simulink library "TemperatureControlLibrary"  (R2024a)
settings: Solver=VariableStepAuto  StartTime=0.0  StopTime=10.0  RelTol=1e-3
undefined symbols (not defined in the file): delay_s, wn, zetaK
libraries: LumArduinoMAX31856 x1, arduinolib x1
settings Model: Creator=chris  LastModifiedBy=chris

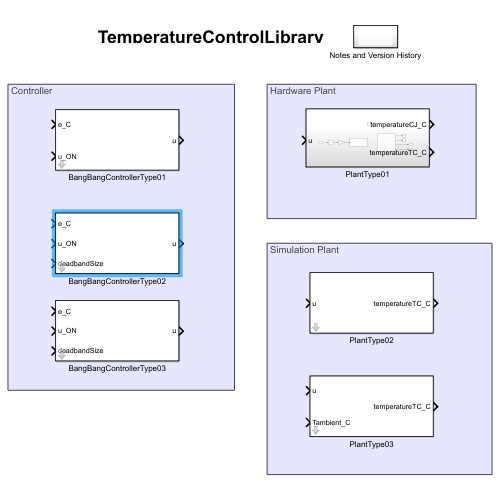
[thumbnail: Simulink's stored preview of the top-level diagram]
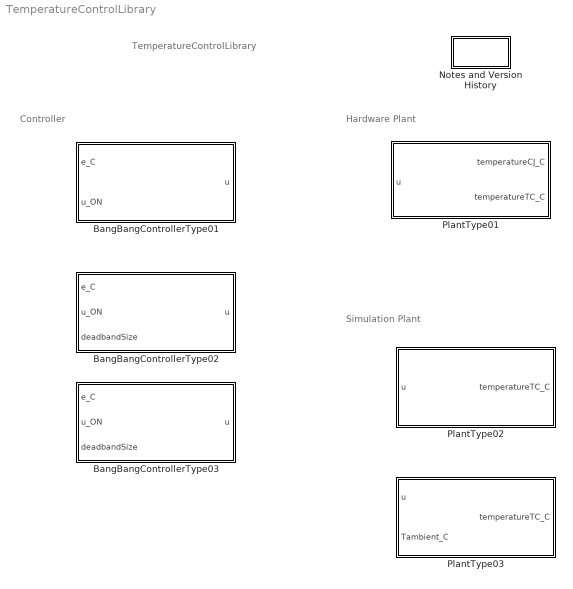
== system TemperatureControlLibrary ==
  note: Simulation Plant
  note: Controller
  note: Hardware Plant
  note: TemperatureControlLibrary
  BangBangControllerType01 : Subsystem
      mask help: Simple bang/bang controller.
  BangBangControllerType02 : Subsystem
      mask help: Bang/bang controller with hysteresis deadband (algorithm is implemented using a memory block).
  BangBangControllerType03 : Subsystem
      mask help: Bang/bang controller with hysteresis deadband (algorithm is implemented as a Stateflow chart).
  Notes and Version History : Subsystem
  PlantType01 : Subsystem
  PlantType02 : Subsystem  mask{a=1, b=1, T0=25}
      mask prompts: T0 "Initial Temperature (C)"
      mask help:
      | Simple first order temperature model
      |
      | DOES NOT APPEAR TO WORK WELL, DO NOT USE
      |
      | Input
      | u = duty cycle (0 = off, 1 = full on)
      |
      | Output
      | temperatureTC_C = temperature (C)
  PlantType03 : Subsystem  mask{wn=wn, zeta=zetaK, K=25, Tdelay_s=delay_s}
      mask prompts: Tdelay_s "Delay time (sec)"
      mask help:
      | Simple first order temperature model
      |
      | Input
      | u = duty cycle (0 = off, 1 = full on)
      |
      | Output
      | temperatureTC_C = temperature (C)

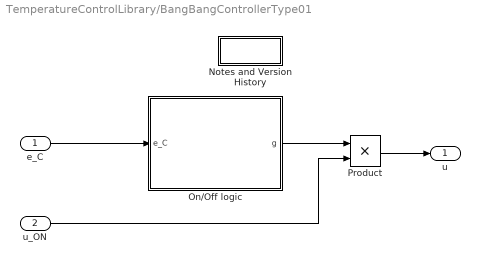
== system TemperatureControlLibrary/BangBangControllerType01 ==
  e_C : Inport
  u_ON : Inport  Port=2
  Notes and Version History : Subsystem
  On/Off logic : MATLAB Function  TreatAsAtomicUnit=on
  Product : Product
  u : Outport
  wires:
  Product/1 -> u/1
  u_ON/1 -> Product/2
  On/Off logic/1(g) -> Product/1
  e_C/1 -> On/Off logic/1(e_C)

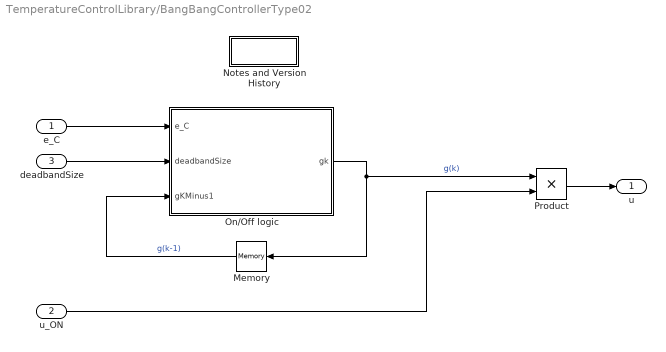
== system TemperatureControlLibrary/BangBangControllerType02 ==
  e_C : Inport
  u_ON : Inport  Port=2
  deadbandSize : Inport  Port=3
  Memory : Memory
  Notes and Version History : Subsystem
  On/Off logic : MATLAB Function  TreatAsAtomicUnit=on
  Product : Product
  u : Outport
  wires:
  e_C/1 -> On/Off logic/1(e_C)
  On/Off logic/1(gk) -> Product/1, Memory/1  "g(k)"
  u_ON/1 -> Product/2
  Product/1 -> u/1
  deadbandSize/1 -> On/Off logic/2(deadbandSize)
  Memory/1 -> On/Off logic/3(gKMinus1)  "g(k-1)"

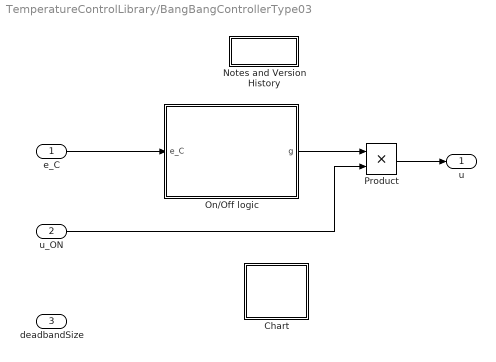
== system TemperatureControlLibrary/BangBangControllerType03 ==
  e_C : Inport
  u_ON : Inport  Port=2
  deadbandSize : Inport  Port=3
  Chart : Stateflow chart  TreatAsAtomicUnit=on
  Notes and Version History : Subsystem
  On/Off logic : MATLAB Function  TreatAsAtomicUnit=on
  Product : Product
  u : Outport
  wires:
  Product/1 -> u/1
  u_ON/1 -> Product/2
  On/Off logic/1(g) -> Product/1
  e_C/1 -> On/Off logic/1(e_C)

== system TemperatureControlLibrary/Notes and Version History ==
  note: Blocks for temperature control.
      |
      | Christopher Lum
      | lum@uw.edu
      |
      | Version History
      | 01/11/25: Created
      | 01/23/25: Adding BangBangControllerType01

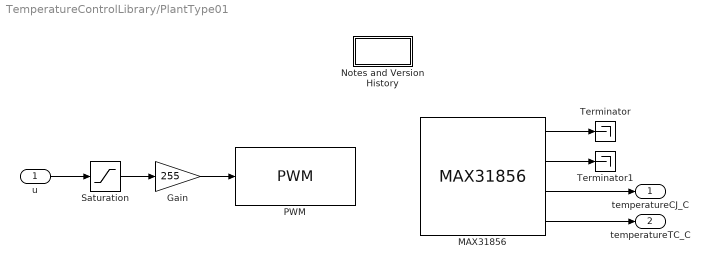
== system TemperatureControlLibrary/PlantType01 ==
  u : Inport
  Gain : Gain  Gain=255
  MAX31856 : LumArduinoMAX31856/MAX31856  MAX31856_CR0_REG_READ=MAX31856_CR0_REG_READ  MAX31856_CR0_REG_WRITE=MAX31856_CR0_REG_WRITE  MAX31856_CR1_REG_READ=MAX31856_CR1_REG_READ  MAX31856_CR1_REG_WRITE=MAX31856_CR1_REG_WRITE  MAX31856_MASK_REG_WRITE=MAX31856_MASK_REG_WRITE  MAX31856_CJTO_REG_READ=MAX31856_CJTO_REG_READ  MAX31856_CJTO_REG_WRITE=MAX31856_CJTO_REG_WRITE  MAX31856_CJTH_REG_READ=MAX31856_CJTH_REG_READ  MAX31856_CJTL_REG_READ=MAX31856_CJTL_REG_READ  MAX31856_LTCBH_REG_READ=MAX31856_LTCBH_REG_READ  MAX31856_LTCBM_REG_READ=MAX31856_LTCBM_REG_READ  MAX31856_LTCBL_REG_READ=MAX31856_LTCBL_REG_READ  deltaT_s=deltaT_s  pin_CS=pin_CS
  Notes and Version History : Subsystem
  PWM : arduinolib/PWM  pinNumber=PinPWM  frequencyType=Default  desiredFrequency=490.2  achievableFrequency=490.2
  Saturation : Saturate  UpperLimit=1  LowerLimit=0
  Terminator : Terminator
  Terminator1 : Terminator
  temperatureCJ_C : Outport
  temperatureTC_C : Outport  Port=2
  wires:
  u/1 -> Saturation/1
  MAX31856/4 -> temperatureTC_C/1
  Gain/1 -> PWM/1
  MAX31856/3 -> temperatureCJ_C/1
  MAX31856/2 -> Terminator1/1
  Saturation/1 -> Gain/1
  MAX31856/1 -> Terminator/1

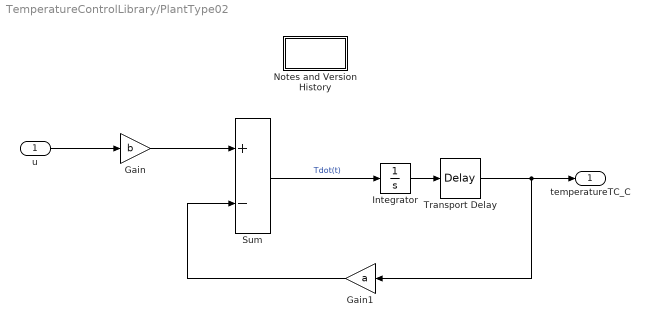
== system TemperatureControlLibrary/PlantType02 ==
  u : Inport
  Gain : Gain  Gain=b
  Gain1 : Gain  Gain=a
  Integrator : Integrator  InitialCondition=T0
  Notes and Version History : Subsystem
  Sum : Sum  Inputs=+-
  Transport Delay : TransportDelay  DelayTime=3
  temperatureTC_C : Outport
  wires:
  u/1 -> Gain/1
  Gain/1 -> Sum/1
  Sum/1 -> Integrator/1  "Tdot(t)"
  Integrator/1 -> Transport Delay/1
  Gain1/1 -> Sum/2
  Transport Delay/1 -> temperatureTC_C/1, Gain1/1

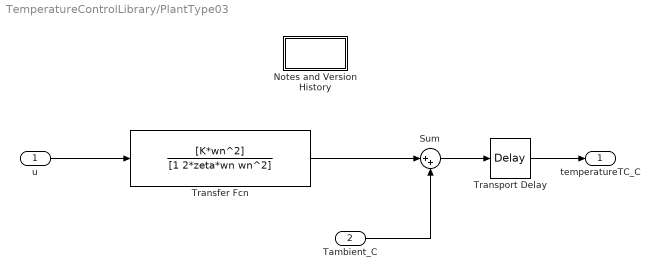
== system TemperatureControlLibrary/PlantType03 ==
  u : Inport
  Tambient_C : Inport  Port=2
  Notes and Version History : Subsystem
  Sum : Sum  Inputs=|++
  Transfer Fcn : TransferFcn  Numerator=[K*wn^2]  Denominator=[1 2*zeta*wn wn^2]
  Transport Delay : TransportDelay  DelayTime=Tdelay_s
  temperatureTC_C : Outport
  wires:
  u/1 -> Transfer Fcn/1
  Tambient_C/1 -> Sum/2
  Sum/1 -> Transport Delay/1
  Transfer Fcn/1 -> Sum/1
  Transport Delay/1 -> temperatureTC_C/1

== system TemperatureControlLibrary/BangBangControllerType01/Notes and Version History ==
  note: Christopher Lum
      | lum@uw.edu
      |
      | Version History
      | 01/24/25: Created

== system TemperatureControlLibrary/BangBangControllerType02/Notes and Version History ==
  note: Christopher Lum
      | lum@uw.edu
      |
      | Version History
      | 01/26/25: Created

== system TemperatureControlLibrary/BangBangControllerType03/Notes and Version History ==
  note: Christopher Lum
      | lum@uw.edu
      |
      | Version History
      | 01/26/25: Created

== system TemperatureControlLibrary/PlantType01/Notes and Version History ==
  note: Christopher Lum
      | lum@uw.edu
      |
      | Version History
      | 01/11/25: Created

== system TemperatureControlLibrary/PlantType02/Notes and Version History ==
  note: Plant used for simulation
      |
      | DOES NOT SEEM TO PERFORM WELL
      |
      | Christopher Lum
      | lum@uw.edu
      |
      | Version History
      | 01/23/25: Created

== system TemperatureControlLibrary/PlantType03/Notes and Version History ==
  note: Plant used for simulation
      |
      | Christopher Lum
      | lum@uw.edu
      |
      | Version History
      | 01/24/25: Created

== matlab function TemperatureControlLibrary/BangBangControllerType02/On//Off logic ==
  data: e_C input; gk output; deadbandSize input; gKMinus1 input
function gk = fcn(e_C, deadbandSize, gKMinus1)

if(e_C > deadbandSize)
    %Turn control on
    gk = 1;
elseif(e < -deadbandSize)
    %Turn control off
    gk = 0;

else
    %in hysteresis band (e in range [-deadbandSize,deadbandSize]
    if(gKMinus1==0)
        gk = 0;
    else
        gk = 1;
    end
end

== matlab function TemperatureControlLibrary/BangBangControllerType01/On//Off logic ==
  data: e_C input; g output
function g = fcn(e_C)

if(e_C > 0)
    %Too cold, turn heater on
    g = 1;
else
    %Too hot, turn heater off
    g = 0;
end

== stateflow chart TemperatureControlLibrary/BangBangControllerType03/Chart ==

== matlab function TemperatureControlLibrary/BangBangControllerType03/On//Off logic ==
  data: e_C input; g output
function g = fcn(e_C)

if(e_C > 0)
    %Too cold, turn heater on
    g = 1;
else
    %Too hot, turn heater off
    g = 0;
end
